simulink model "motoman_enghouse"  (Simulink 6.2)
settings: Solver=ode45  SolverMode=SingleTasking  StartTime=0.0  StopTime=10.0  RelTol=1e-3  AbsTol=1e-6
settings Model: Creator=The MathWorks Inc.  LastModifiedBy=suarezjl  ExtModeTrigMode=oneshot  ExtModeArmWhenConnect=off  ExtModeAutoUpdateStatusClock=off
settings DataIOCC: LimitDataPoints=off  SignalLoggingName=logsOut
settings OptimizationCC: BooleanDataType=off  InlineInvariantSignals=on
settings DebuggingCC: CheckExecutionContextPreStartOutputMsg=on  CheckExecutionContextRuntimeOutputMsg=on  IntegerOverflowMsg=none
settings HardwareCC: TargetUnknown=on
settings ModelReferenceCC: UpdateModelReferenceTargets=IfOutOfDate

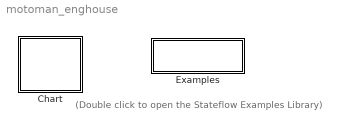
== system motoman_enghouse ==
  note: (Double click to open the
      | Stateflow Examples Library)
  Chart : Stateflow chart
  Examples : Subsystem
      settings: OpenFcn=sf('Private','sf_examples')
      mask Display: disp('Examples')

== system motoman_enghouse/Examples ==

== stateflow chart Chart ==
  state //Initialize
    Aquateen\MotomanArm\HP3JC.connect_Initialize()
    Aquateen\MotomanArm\HP3JC.servo_ServoOn()
    Aquateen\MotomanArm\StateMachine.Wait(500)
  state //RunJob
    Aquateen\MotomanArm\HP3JC.job_CopyTextQueue()
    Aquateen\MotomanArm\HP3JC.job_SelectJob()
    Aquateen\MotomanArm\HP3JC.job_StartJob()
    Aquateen\MotomanArm\StateMachine.Wait(500)
    Aquateen\MotomanArm\HP3JC.job_StartJob()
  state //Close BarretHand
    Aquateen\MotomanArm\BarretHand.Close()
    Aquateen\MotomanArm\StateMachine.Wait(1000)
  state //Disconnect
    Aquateen\MotomanArm\HP3JC.connect_Disconnect()
  (default) -> //Initialize : Start
  //Close BarretHand -> //RunJob : Default
  //Initialize -> //Close BarretHand : Default
  //RunJob -> //Disconnect : Signal="Stop"
